simulink model "sum_tones_test"  (R2016b)
settings: Solver=VariableStepAuto  StartTime=0.0  StopTime=2^16/Fadc  RelTol=1e-3  EnableMultiTasking=on
PreLoadFcn:
  | setup
values from neighbouring files (symbols this model uses):
  Fadc = 614.4e6    (= 614400000)    [setup.m]
libraries: xbsIndex_r4 x22, dspsigops x15, simulink x1, CryoDetLibCMB x1
settings Model: Creator=Mitch  LastModifiedBy=mdewart
settings OptimizationCC: LifeSpan=inf
settings DebuggingCC: SFUnexpectedBacktrackingDiag=warning  SFNoUnconditionalDefaultTransitionDiag=warning  SFExecutionAtInitializationDiag=none
settings GRTTargetCC: TargetLangStandard=C89/C90 (ANSI)  GeneratePreprocessorConditionals=Disable all
settings ConfigComp: CovMetricSettings=dw  CovHtmlReporting=on  CovSaveCumulativeToWorkspaceVar=on  CovSaveSingleToWorkspaceVar=on  CovExternalEMLEnable=off

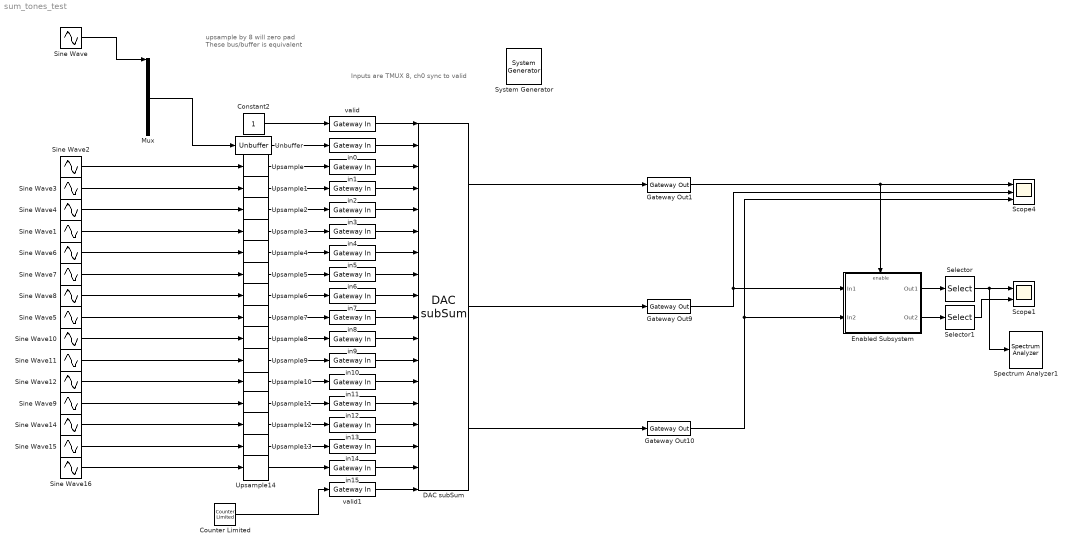
== system sum_tones_test ==
  note: upsample by 8 will zero pad
      | These bus/buffer is equivalent
  note: Inputs are TMUX 8, ch0 sync to valid
  " System Generator" : xbsIndex_r4/ System Generator  Tag=genX  xilinxfamily=kintexu  part=xcku040  speed=-2-e  package=ffva1156  synthesis_tool=Vivado  clock_wrapper=Clock Enables  directory=./netlist  proj_type=Vivado  Synth_file=Vivado Synthesis Defaults  Impl_file=Vivado Implementation Defaults  testbench=off  simulink_period=2/Fadc  sysclk_period=2e9/Fadc  dcm_input_clock_period=10  incr_netlist=off  trim_vbits=Everywhere in SubSystem  dbl_ovrd=According to Block Masks  core_generation=According to Block Masks  run_coregen=off  deprecated_control=off  eval_field=0  block_type=sysgen
  Constant2 : Constant  SampleTime=2/Fadc
  Counter Limited : simulink/Sources/Counter Limited  uplimit=7  tsamp=2/Fadc
  DAC subSum : CryoDetLibCMB/DAC subSum
  Enabled Subsystem : Subsystem  TreatAsAtomicUnit=on
  Gateway Out1 : xbsIndex_r4/Gateway Out  inherit_from_input=off  hdl_port=on  rows=1  columns=1  UseAsDAC=off  DACChannel='1'  interface=None  automatic_assignment=on  address_offset=hex2dec('00')  intf_name=''  intf_description=''  timing_constraint=None  locs_specified=off  LOCs={}  io_standard={}  block_type=gatewayout
  Gateway Out10 : xbsIndex_r4/Gateway Out  inherit_from_input=off  hdl_port=on  rows=1  columns=1  UseAsDAC=off  DACChannel='1'  interface=None  automatic_assignment=on  address_offset=hex2dec('00')  intf_name=''  intf_description=''  timing_constraint=None  locs_specified=off  LOCs={}  io_standard={}  block_type=gatewayout
  Gateway Out9 : xbsIndex_r4/Gateway Out  inherit_from_input=off  hdl_port=on  rows=1  columns=1  UseAsDAC=off  DACChannel='1'  interface=None  automatic_assignment=on  address_offset=hex2dec('00')  intf_name=''  intf_description=''  timing_constraint=None  locs_specified=off  LOCs={}  io_standard={}  block_type=gatewayout
  Mux : Mux  Inputs=8
  Scope1 : Scope  NumInputPorts=2
  Scope4 : Scope  NumInputPorts=3
  Selector : Selector  InputPortWidth=8  IndexOptions=Index vector (dialog)  Indices=[1]  OutputSizes=1
  Selector1 : Selector  InputPortWidth=8  IndexOptions=Index vector (dialog)  Indices=[1]  OutputSizes=1
  Sine Wave : Sin  Frequency=2*pi*5.2e6  SampleTime=16/Fadc
  Sine Wave1 : Sin  Frequency=2*pi*(4+randn(1))*1e6  SampleTime=16/Fadc
  Sine Wave10 : Sin  Frequency=2*pi*(12+randn(1))*1e6  SampleTime=16/Fadc
  Sine Wave11 : Sin  Frequency=2*pi*(14+randn(1))*1e6  SampleTime=16/Fadc
  Sine Wave12 : Sin  Frequency=2*pi*(16+randn(1))*1e6  SampleTime=16/Fadc
  Sine Wave14 : Sin  Frequency=2*pi*(20+randn(1))*1e6  SampleTime=16/Fadc
  Sine Wave15 : Sin  Frequency=2*pi*(22+randn(1))*1e6  SampleTime=16/Fadc
  Sine Wave16 : Sin  Frequency=2*pi*(24+randn(1))*1e6  SampleTime=16/Fadc
  Sine Wave2 : Sin  Frequency=2*pi*(2+randn(1))*1e6  SampleTime=16/Fadc
  Sine Wave3 : Sin  Frequency=2*pi*(3+randn(1))*1e6  SampleTime=16/Fadc
  Sine Wave4 : Sin  Frequency=2*pi*(4+randn(1))*1e6  SampleTime=16/Fadc
  Sine Wave5 : Sin  Frequency=2*pi*(10+randn(1))*1e6  SampleTime=16/Fadc
  Sine Wave6 : Sin  Frequency=2*pi*(5+randn(1))*1e6  SampleTime=16/Fadc
  Sine Wave7 : Sin  Frequency=2*pi*(6+randn(1))*1e6  SampleTime=16/Fadc
  Sine Wave8 : Sin  Frequency=2*pi*(8+randn(1))*1e6  SampleTime=16/Fadc
  Sine Wave9 : Sin  Frequency=2*pi*(18+randn(1))*1e6  SampleTime=16/Fadc
  Spectrum Analyzer1 : SpectrumAnalyzer
  Unbuffer : Unbuffer  SampleBasedProcessing=Same as frame based
  Upsample{,1..14} (15 alike) : dspsigops/Upsample  N=8  phase=0  RateOptions=Allow multirate processing  ic=0  mode=Unused parameter value
  in{0..15} (16 alike) : xbsIndex_r4/Gateway In  gui_display_data_type=Fixed-point  arith_type="Signed  (2's comp)"  n_bits=16  bin_pt=15  preci_type=Single  exp_width=8  frac_width=24  rows=1  columns=1  quantization="Round  (unbiased: +/- Inf)"  overflow=Saturate  period=2/Fadc  UseAsADC=off  ADCChannel='1'  interface=None  automatic_assignment=on  address_offset=hex2dec('00')  intf_name=''  intf_description=''  default_value=0  timing_constraint=None  locs_specified=off  LOCs={}  io_standard={}  inherit_from_input=off  hdl_port=on  dbl_ovrd=off  block_type=gatewayin
  valid : xbsIndex_r4/Gateway In  gui_display_data_type=Boolean  arith_type=Boolean  n_bits=18  bin_pt=15  preci_type=Single  exp_width=8  frac_width=24  rows=1  columns=1  quantization="Round  (unbiased: +/- Inf)"  overflow=Saturate  period=2/Fadc  UseAsADC=off  ADCChannel='1'  interface=None  automatic_assignment=on  address_offset=hex2dec('00')  intf_name=''  intf_description=''  default_value=0  timing_constraint=None  locs_specified=off  LOCs={}  io_standard={}  inherit_from_input=off  hdl_port=on  dbl_ovrd=off  block_type=gatewayin
  valid1 : xbsIndex_r4/Gateway In  gui_display_data_type=Fixed-point  arith_type=Unsigned  n_bits=3  bin_pt=0  preci_type=Single  exp_width=8  frac_width=24  rows=1  columns=1  quantization="Round  (unbiased: +/- Inf)"  overflow=Saturate  period=2/Fadc  UseAsADC=off  ADCChannel='1'  interface=None  automatic_assignment=on  address_offset=hex2dec('00')  intf_name=''  intf_description=''  default_value=0  timing_constraint=None  locs_specified=off  LOCs={}  io_standard={}  inherit_from_input=off  hdl_port=on  dbl_ovrd=off  block_type=gatewayin
  wires:
  Constant2/1 -> valid/1
  Mux/1 -> Unbuffer/1
  Unbuffer/1 -> in0/1
  DAC subSum/2 -> Gateway Out9/1
  DAC subSum/3 -> Gateway Out10/1
  DAC subSum/1 -> Gateway Out1/1
  Gateway Out9/1 -> Scope4/2, Enabled Subsystem/1(In1)
  Gateway Out10/1 -> Scope4/3, Enabled Subsystem/2(In2)
  Sine Wave/1 -> Mux/1
  valid1/1 -> DAC subSum/18
  Counter Limited/1 -> valid1/1
  Gateway Out1/1 -> Enabled Subsystem/Enable, Scope4/1
  Enabled Subsystem/1(Out1) -> Selector/1
  Selector/1 -> Scope1/1, Spectrum Analyzer1/1
  Sine Wave2/1 -> Upsample/1
  Sine Wave3/1 -> Upsample1/1
  Sine Wave4/1 -> Upsample2/1
  Sine Wave1/1 -> Upsample3/1
  Sine Wave6/1 -> Upsample4/1
  Sine Wave7/1 -> Upsample5/1
  Sine Wave8/1 -> Upsample6/1
  Sine Wave5/1 -> Upsample7/1
  Upsample/1 -> in1/1
  Upsample1/1 -> in2/1
  Upsample2/1 -> in3/1
  Upsample3/1 -> in4/1
  Upsample4/1 -> in5/1
  Upsample5/1 -> in6/1
  Upsample6/1 -> in7/1
  Upsample7/1 -> in8/1
  Sine Wave10/1 -> Upsample8/1
  Sine Wave11/1 -> Upsample9/1
  Sine Wave12/1 -> Upsample10/1
  Sine Wave9/1 -> Upsample11/1
  Sine Wave14/1 -> Upsample12/1
  Sine Wave15/1 -> Upsample13/1
  Sine Wave16/1 -> Upsample14/1
  Upsample8/1 -> in9/1
  Upsample9/1 -> in10/1
  Upsample10/1 -> in11/1
  Upsample11/1 -> in12/1
  Upsample12/1 -> in13/1
  Upsample13/1 -> in14/1
  Upsample14/1 -> in15/1
  in3/1 -> DAC subSum/5
  in4/1 -> DAC subSum/6
  in6/1 -> DAC subSum/8
  in11/1 -> DAC subSum/13
  in8/1 -> DAC subSum/10
  valid/1 -> DAC subSum/1
  in0/1 -> DAC subSum/2
  in14/1 -> DAC subSum/16
  in7/1 -> DAC subSum/9
  in2/1 -> DAC subSum/4
  in5/1 -> DAC subSum/7
  in10/1 -> DAC subSum/12
  in12/1 -> DAC subSum/14
  in1/1 -> DAC subSum/3
  in9/1 -> DAC subSum/11
  in15/1 -> DAC subSum/17
  in13/1 -> DAC subSum/15
  Selector1/1 -> Scope1/2
  Enabled Subsystem/2(Out2) -> Selector1/1

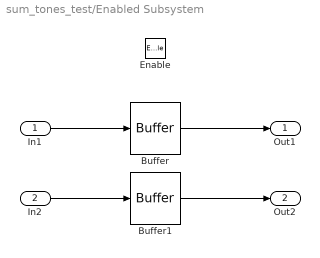
== system sum_tones_test/Enabled Subsystem ==
  In1 : Inport
  In2 : Inport  Port=2
  Enable : EnablePort
  Buffer : Buffer  N=8  TreatMby1Signals=One channel  OutputFrames=off
  Buffer1 : Buffer  N=8  TreatMby1Signals=One channel  OutputFrames=off
  Out1 : Outport
  Out2 : Outport  Port=2
  wires:
  In1/1 -> Buffer/1
  Buffer/1 -> Out1/1
  In2/1 -> Buffer1/1
  Buffer1/1 -> Out2/1
